simulink model "motor_float_open_loop_model"  (R2023b)
settings: Solver=FixedStepDiscrete  StartTime=0.0  StopTime=simcfg.stop_time  FixedStep=simcfg.Ts_plant  RelTol=1e-3
undefined symbols (not defined in the file or in its folder): inverter, motor, openloop, simcfg
libraries: mcbplantlib x1, autolibpmsmexterior x1
settings Model: DataDictionary=motor_float_interface.sldd  Creator=user  LastModifiedBy=user
settings OptimizationCC: DefaultParameterBehavior=Inlined  EnhancedBackFolding=on  PassReuseOutputArgsAs=Individual arguments  OptimizeBlockOrder=speed  DifferentSizesBufferReuse=on  OptimizationCustomize=off  EfficientTunableParamExpr=on
settings DebuggingCC: ParameterTunabilityLossMsg=error
settings HardwareCC: ProdBitPerPointer=32  ProdBitPerSizeT=32  ProdBitPerPtrDiffT=32  ProdLargestAtomicInteger=Long  ProdLargestAtomicFloat=Double  ProdWordSize=32  ProdHWDeviceType=ARM Compatible->ARM Cortex  TargetLargestAtomicInteger=Long  TargetLargestAtomicFloat=Double  TargetIntDivRoundTo=Zero  TargetEndianess=LittleEndian  TargetHWDeviceType=ARM Compatible->ARM Cortex  ProdEqTarget=off
settings SFSimCC: MATLABDynamicMemAlloc=off
settings RTWCC: Description=Embedded Coder  SystemTargetFile=ert.tlc  GenCodeOnly=on  TemplateMakefile=ert_default_tmf  GenerateReport=on
settings CodeAppCC: ForceParamTrailComments=on  IgnoreCustomStorageClasses=off  OperatorAnnotations=on  SimulinkDataObjDesc=on  SFDataObjDesc=on  InsertBlockDesc=on
settings ERTTargetCC: TargetLangStandard=C99 (ISO)  CodeInterfacePackaging=Reusable function  InlinedParameterPlacement=NonHierarchical  ERTCustomFileTemplate=example_file_process.tlc

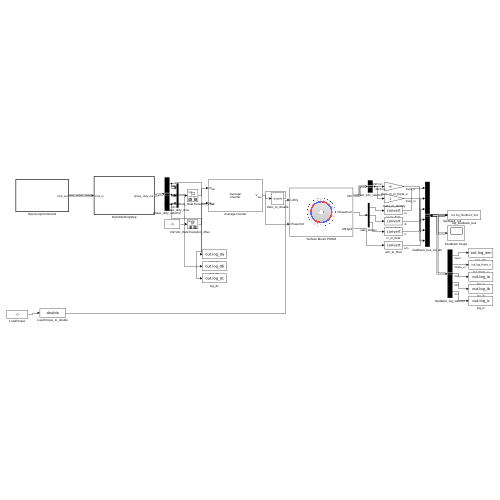
[thumbnail: Simulink's stored preview of the top-level diagram]
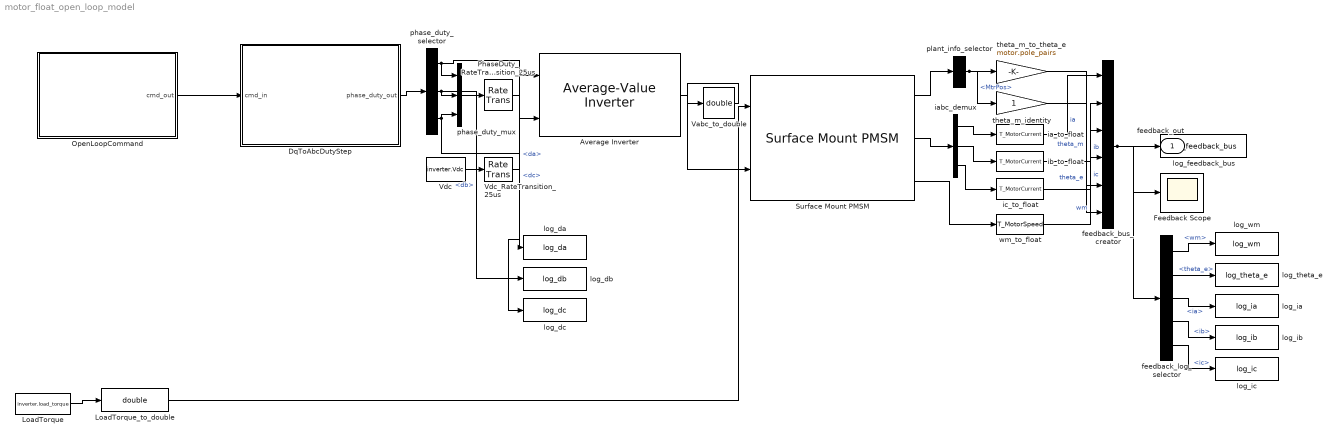
== system motor_float_open_loop_model ==
  Average Inverter : mcbplantlib/Average-Value Inverter
  DqToAbcDutyStep : Subsystem  TreatAsAtomicUnit=on  RTWFcnName=DqToAbcDutyStep  RTWFileName=DqToAbcDutyStep
      settings: RTWFcnNameOpts=User specified  RTWFileNameOpts=User specified
  Feedback Scope : Scope
  LoadTorque : Constant  Value=inverter.load_torque  OutDataTypeStr=T_MotorTorque  SampleTime=simcfg.Ts_plant
  LoadTorque_to_double : DataTypeConversion  OutDataTypeStr=double  SaturateOnIntegerOverflow=off  RndMeth=Floor
  OpenLoopCommand : Subsystem  TreatAsAtomicUnit=on  RTWFcnName=OpenLoopCommandStep  RTWFileName=OpenLoopCommandStep
      settings: RTWFcnNameOpts=User specified  RTWFileNameOpts=User specified
  PhaseDuty_RateTransition_25us : RateTransition  OutPortSampleTime=simcfg.Ts_plant
  Surface Mount PMSM : autolibpmsmexterior/Surface Mount PMSM  port_config=Torque  sim_type=Discrete  Ts=simcfg.Ts_plant  P=motor.pole_pairs  Rs=motor.Rs  Ldq_=motor.Ld  KConstText=Permanent flux linkage constant (lambda_pm):  lambda_pm=motor.psi_f  Ke=159.9771  Kt=1.323  mechanical=[motor.J, motor.B, 0]  idq0=[0 0]  theta_init=0  omega_init=0  KConst=motor.psi_f  lambda_pm_calc=motor.psi_f  RefBlkName='autolibpmsmexterior/Surface Mount PMSM'  aMode=5  Ldq="[0.0017      0.0017]"
  Vabc_to_double : DataTypeConversion  OutDataTypeStr=double  SaturateOnIntegerOverflow=off  RndMeth=Floor
  Vdc : Constant  Value=inverter.Vdc  OutDataTypeStr=T_MotorVoltage  SampleTime=simcfg.Ts_plant
  Vdc_RateTransition_25us : RateTransition  OutPortSampleTime=simcfg.Ts_plant
  feedback_bus_creator : BusCreator  Inputs=6  OutDataTypeStr=Bus: plant_feedback_t  NonVirtualBus=on
  feedback_log_selector : BusSelector  OutputSignals=wm,theta_e,ia,ib,ic
  ia_to_float : DataTypeConversion  OutDataTypeStr=T_MotorCurrent  SaturateOnIntegerOverflow=off  RndMeth=Floor
  iabc_demux : Demux  Outputs=3
  ib_to_float : DataTypeConversion  OutDataTypeStr=T_MotorCurrent  SaturateOnIntegerOverflow=off  RndMeth=Floor
  ic_to_float : DataTypeConversion  OutDataTypeStr=T_MotorCurrent  SaturateOnIntegerOverflow=off  RndMeth=Floor
  log_da : ToWorkspace  VariableName=log_da  SaveFormat=Timeseries  SampleTime=-1
  log_db : ToWorkspace  VariableName=log_db  SaveFormat=Timeseries  SampleTime=-1
  log_dc : ToWorkspace  VariableName=log_dc  SaveFormat=Timeseries  SampleTime=-1
  log_feedback_bus : ToWorkspace  VariableName=log_feedback_bus  SaveFormat=Timeseries  SampleTime=-1
  log_ia : ToWorkspace  VariableName=log_ia  SaveFormat=Timeseries  SampleTime=-1
  log_ib : ToWorkspace  VariableName=log_ib  SaveFormat=Timeseries  SampleTime=-1
  log_ic : ToWorkspace  VariableName=log_ic  SaveFormat=Timeseries  SampleTime=-1
  log_theta_e : ToWorkspace  VariableName=log_theta_e  SaveFormat=Timeseries  SampleTime=-1
  log_wm : ToWorkspace  VariableName=log_wm  SaveFormat=Timeseries  SampleTime=-1
  phase_duty_mux : Mux  Inputs=3
  phase_duty_selector : BusSelector  OutputSignals=da,db,dc
  plant_info_selector : BusSelector  OutputSignals=MtrPos
  theta_m_identity : Gain  OutDataTypeStr=T_MotorAngle
  theta_m_to_theta_e : Gain  Gain=motor.pole_pairs  OutDataTypeStr=T_MotorAngle
  wm_to_float : DataTypeConversion  OutDataTypeStr=T_MotorSpeed  SaturateOnIntegerOverflow=off  RndMeth=Floor
  feedback_out : Outport  OutDataTypeStr=Bus: plant_feedback_t
  wires:
  OpenLoopCommand/1(cmd_out) -> DqToAbcDutyStep/1(cmd_in)
  DqToAbcDutyStep/1(phase_duty_out) -> phase_duty_selector/1
  phase_duty_selector/1 -> phase_duty_mux/1, log_da/1  "<da>"
  phase_duty_selector/2 -> phase_duty_mux/2, log_db/1  "<db>"
  phase_duty_selector/3 -> phase_duty_mux/3, log_dc/1  "<dc>"
  phase_duty_mux/1 -> PhaseDuty_RateTransition_25us/1
  PhaseDuty_RateTransition_25us/1 -> Average Inverter/1
  Vdc/1 -> Vdc_RateTransition_25us/1
  Vdc_RateTransition_25us/1 -> Average Inverter/2
  LoadTorque/1 -> LoadTorque_to_double/1
  LoadTorque_to_double/1 -> Surface Mount PMSM/1
  Average Inverter/1 -> Vabc_to_double/1
  Vabc_to_double/1 -> Surface Mount PMSM/2
  Surface Mount PMSM/1 -> plant_info_selector/1
  plant_info_selector/1 -> theta_m_to_theta_e/1, theta_m_identity/1  "<MtrPos>"
  Surface Mount PMSM/2 -> iabc_demux/1
  iabc_demux/1 -> ia_to_float/1
  iabc_demux/2 -> ib_to_float/1
  iabc_demux/3 -> ic_to_float/1
  Surface Mount PMSM/3 -> wm_to_float/1
  ia_to_float/1 -> feedback_bus_creator/1  "ia"
  ib_to_float/1 -> feedback_bus_creator/2  "ib"
  ic_to_float/1 -> feedback_bus_creator/3  "ic"
  wm_to_float/1 -> feedback_bus_creator/4  "wm"
  theta_m_identity/1 -> feedback_bus_creator/5  "theta_m"
  theta_m_to_theta_e/1 -> feedback_bus_creator/6  "theta_e"
  feedback_bus_creator/1 -> feedback_out/1, log_feedback_bus/1, Feedback Scope/1, feedback_log_selector/1
  feedback_log_selector/1 -> log_wm/1  "<wm>"
  feedback_log_selector/2 -> log_theta_e/1  "<theta_e>"
  feedback_log_selector/3 -> log_ia/1  "<ia>"
  feedback_log_selector/4 -> log_ib/1  "<ib>"
  feedback_log_selector/5 -> log_ic/1  "<ic>"

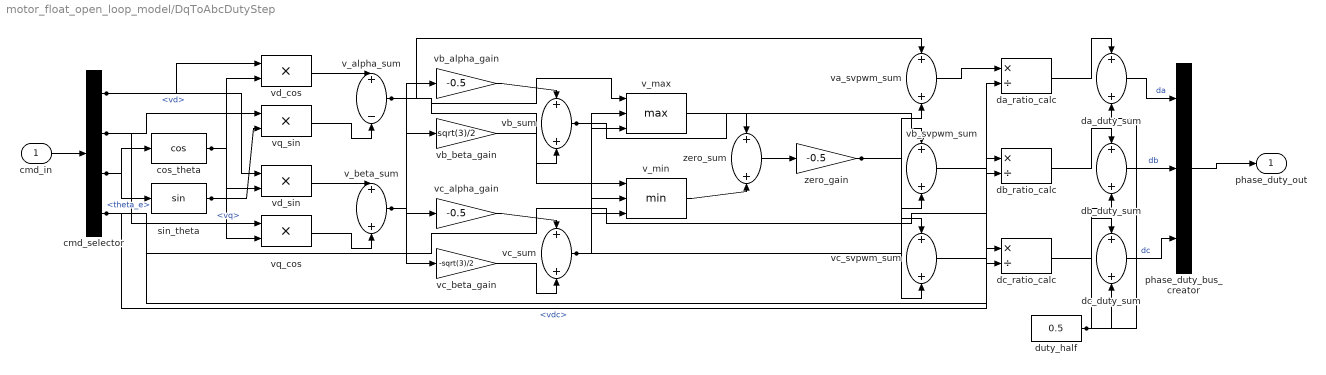
== system motor_float_open_loop_model/DqToAbcDutyStep ==
  cmd_in : Inport  OutDataTypeStr=Bus: open_loop_cmd_t  BusOutputAsStruct=on
  cmd_selector : BusSelector  OutputSignals=vd,vq,theta_e,vdc
  cos_theta : Trigonometry  Operator=cos
  da_duty_sum : Sum  OutDataTypeStr=T_DutyRatio  AccumDataTypeStr=T_DutyRatio
  da_ratio_calc : Product  Inputs=*/  OutDataTypeStr=T_DutyRatio
  db_duty_sum : Sum  OutDataTypeStr=T_DutyRatio  AccumDataTypeStr=T_DutyRatio
  db_ratio_calc : Product  Inputs=*/  OutDataTypeStr=T_DutyRatio
  dc_duty_sum : Sum  OutDataTypeStr=T_DutyRatio  AccumDataTypeStr=T_DutyRatio
  dc_ratio_calc : Product  Inputs=*/  OutDataTypeStr=T_DutyRatio
  duty_half : Constant  Value=0.5  OutDataTypeStr=T_DutyRatio  SampleTime=simcfg.Ts_ctrl
  phase_duty_bus_creator : BusCreator  Inputs=3  OutDataTypeStr=Bus: phase_duty_t  NonVirtualBus=on
  sin_theta : Trigonometry
  v_alpha_sum : Sum  Inputs=+-  OutDataTypeStr=T_MotorVoltage  AccumDataTypeStr=T_MotorVoltage
  v_beta_sum : Sum  OutDataTypeStr=T_MotorVoltage  AccumDataTypeStr=T_MotorVoltage
  v_max : MinMax  Function=max  Inputs=3
  v_min : MinMax  Inputs=3
  va_svpwm_sum : Sum  OutDataTypeStr=T_MotorVoltage  AccumDataTypeStr=T_MotorVoltage
  vb_alpha_gain : Gain  Gain=-0.5  ParamDataTypeStr=T_MotorFloat  OutDataTypeStr=T_MotorVoltage
  vb_beta_gain : Gain  Gain=sqrt(3)/2  ParamDataTypeStr=T_MotorFloat  OutDataTypeStr=T_MotorVoltage
  vb_sum : Sum  OutDataTypeStr=T_MotorVoltage  AccumDataTypeStr=T_MotorVoltage
  vb_svpwm_sum : Sum  OutDataTypeStr=T_MotorVoltage  AccumDataTypeStr=T_MotorVoltage
  vc_alpha_gain : Gain  Gain=-0.5  ParamDataTypeStr=T_MotorFloat  OutDataTypeStr=T_MotorVoltage
  vc_beta_gain : Gain  Gain=-sqrt(3)/2  ParamDataTypeStr=T_MotorFloat  OutDataTypeStr=T_MotorVoltage
  vc_sum : Sum  OutDataTypeStr=T_MotorVoltage  AccumDataTypeStr=T_MotorVoltage
  vc_svpwm_sum : Sum  OutDataTypeStr=T_MotorVoltage  AccumDataTypeStr=T_MotorVoltage
  vd_cos : Product  Inputs=**  OutDataTypeStr=T_MotorVoltage
  vd_sin : Product  Inputs=**  OutDataTypeStr=T_MotorVoltage
  vq_cos : Product  Inputs=**  OutDataTypeStr=T_MotorVoltage
  vq_sin : Product  Inputs=**  OutDataTypeStr=T_MotorVoltage
  zero_gain : Gain  Gain=-0.5  ParamDataTypeStr=T_MotorFloat  OutDataTypeStr=T_MotorVoltage
  zero_sum : Sum  OutDataTypeStr=T_MotorVoltage  AccumDataTypeStr=T_MotorVoltage
  phase_duty_out : Outport  OutDataTypeStr=Bus: phase_duty_t
  wires:
  cmd_in/1 -> cmd_selector/1
  cmd_selector/3 -> cos_theta/1, sin_theta/1  "<theta_e>"
  cmd_selector/1 -> vd_cos/1, vd_sin/1  "<vd>"
  cos_theta/1 -> vd_cos/2, vq_cos/2
  cmd_selector/2 -> vq_sin/1, vq_cos/1  "<vq>"
  sin_theta/1 -> vq_sin/2, vd_sin/2
  vd_cos/1 -> v_alpha_sum/1
  vq_sin/1 -> v_alpha_sum/2
  vd_sin/1 -> v_beta_sum/1
  vq_cos/1 -> v_beta_sum/2
  v_alpha_sum/1 -> vb_alpha_gain/1, vc_alpha_gain/1, v_max/1, v_min/1, va_svpwm_sum/1
  v_beta_sum/1 -> vb_beta_gain/1, vc_beta_gain/1
  vb_alpha_gain/1 -> vb_sum/1
  vb_beta_gain/1 -> vb_sum/2
  vc_alpha_gain/1 -> vc_sum/1
  vc_beta_gain/1 -> vc_sum/2
  vb_sum/1 -> v_max/2, v_min/2, vb_svpwm_sum/1
  vc_sum/1 -> v_max/3, v_min/3, vc_svpwm_sum/1
  v_max/1 -> zero_sum/1
  v_min/1 -> zero_sum/2
  zero_sum/1 -> zero_gain/1
  zero_gain/1 -> va_svpwm_sum/2, vb_svpwm_sum/2, vc_svpwm_sum/2
  va_svpwm_sum/1 -> da_ratio_calc/1
  cmd_selector/4 -> da_ratio_calc/2, db_ratio_calc/2, dc_ratio_calc/2  "<vdc>"
  vb_svpwm_sum/1 -> db_ratio_calc/1
  vc_svpwm_sum/1 -> dc_ratio_calc/1
  da_ratio_calc/1 -> da_duty_sum/1
  db_ratio_calc/1 -> db_duty_sum/1
  dc_ratio_calc/1 -> dc_duty_sum/1
  duty_half/1 -> da_duty_sum/2, db_duty_sum/2, dc_duty_sum/2
  da_duty_sum/1 -> phase_duty_bus_creator/1  "da"
  db_duty_sum/1 -> phase_duty_bus_creator/2  "db"
  dc_duty_sum/1 -> phase_duty_bus_creator/3  "dc"
  phase_duty_bus_creator/1 -> phase_duty_out/1

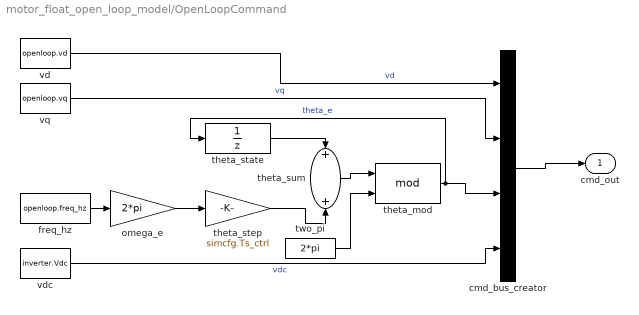
== system motor_float_open_loop_model/OpenLoopCommand ==
  cmd_bus_creator : BusCreator  Inputs=4  OutDataTypeStr=Bus: open_loop_cmd_t  NonVirtualBus=on
  freq_hz : Constant  Value=openloop.freq_hz  OutDataTypeStr=T_MotorFloat  SampleTime=simcfg.Ts_ctrl
  omega_e : Gain  Gain=2*pi  ParamDataTypeStr=T_MotorFloat  OutDataTypeStr=T_MotorFloat
  theta_mod : Math  Operator=mod  OutDataTypeStr=T_MotorAngle
  theta_state : UnitDelay  SampleTime=simcfg.Ts_ctrl  HasFrameUpgradeWarning=on
  theta_step : Gain  Gain=simcfg.Ts_ctrl  ParamDataTypeStr=T_MotorFloat  OutDataTypeStr=T_MotorAngle
  theta_sum : Sum  OutDataTypeStr=T_MotorAngle  AccumDataTypeStr=T_MotorAngle
  two_pi : Constant  Value=2*pi  OutDataTypeStr=T_MotorAngle  SampleTime=simcfg.Ts_ctrl
  vd : Constant  Value=openloop.vd  OutDataTypeStr=T_MotorVoltage  SampleTime=simcfg.Ts_ctrl
  vdc : Constant  Value=inverter.Vdc  OutDataTypeStr=T_MotorVoltage  SampleTime=simcfg.Ts_ctrl
  vq : Constant  Value=openloop.vq  OutDataTypeStr=T_MotorVoltage  SampleTime=simcfg.Ts_ctrl
  cmd_out : Outport  OutDataTypeStr=Bus: open_loop_cmd_t
  wires:
  freq_hz/1 -> omega_e/1
  omega_e/1 -> theta_step/1
  theta_state/1 -> theta_sum/1
  theta_step/1 -> theta_sum/2
  theta_sum/1 -> theta_mod/1
  two_pi/1 -> theta_mod/2
  theta_mod/1 -> theta_state/1, cmd_bus_creator/3  "theta_e"
  vd/1 -> cmd_bus_creator/1  "vd"
  vq/1 -> cmd_bus_creator/2  "vq"
  vdc/1 -> cmd_bus_creator/4  "vdc"
  cmd_bus_creator/1 -> cmd_out/1
